simulink model "EV_sim_model"  (R2024a)
settings: Solver=FixedStepAuto  StartTime=0.0  StopTime=time  FixedStep=0.01  RelTol=1e-3
undefined symbols (not defined in the file): Af, Bl, C, Cd, eff_b, eff_g, eff_m, g, GR, Grd, i, Jgb, Jw, L_range, M, pho_air, R_w, U_bat, U_pack
libraries: autolibshared x4
settings Model: Creator=Roshan_PC  LastModifiedBy=Roshan_PC
settings SolverCC: ZeroCrossAlgorithm=Adaptive
settings DebuggingCC: MaskedZcDiagnostic=none  IgnoredZcDiagnostic=none

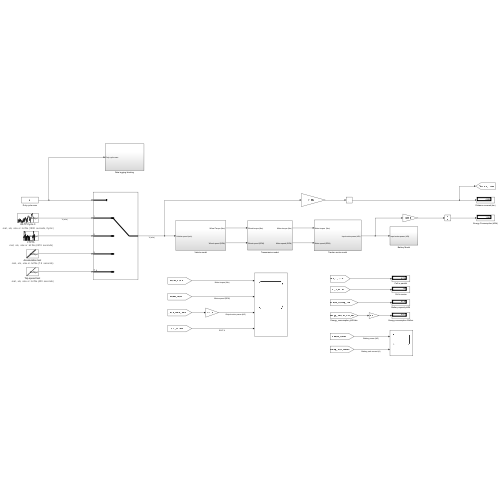
[thumbnail: Simulink's stored preview of the top-level diagram]
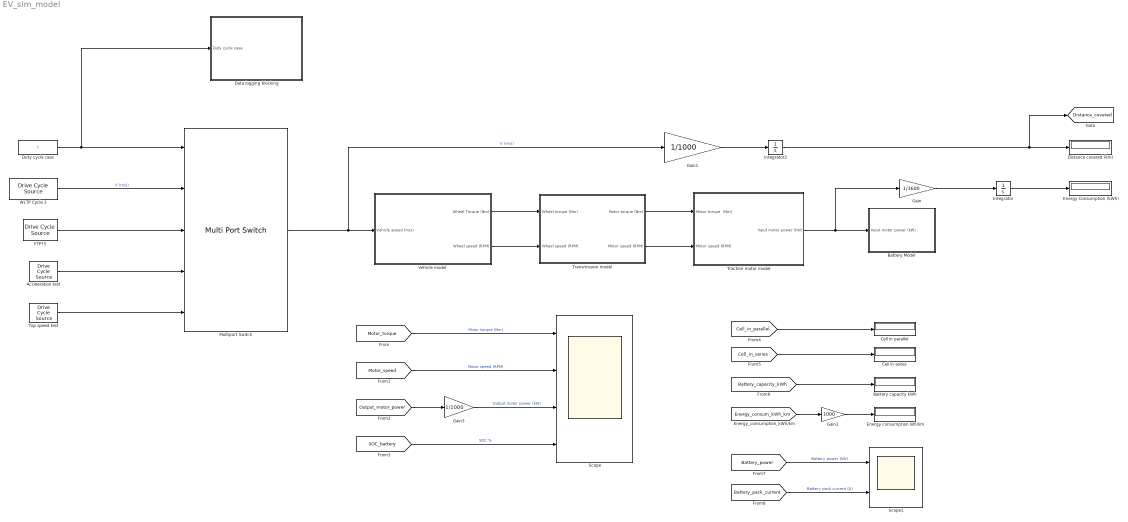
== system EV_sim_model ==
  Acceleration test : autolibshared/Drive Cycle Source  cycleVar=.mat, .xls, .xlsx or .txt file  fileVar=D:\Creation stuff\Academic\MATLAB practice\1_EV_car_system_simulation\Backward_approach\Model-2\Acceleration_Drive_Cycle.xlsx  tfinal="7.9  seconds"  cycleRepeat=off  outAccPort=off  outGearPort=off  gearList=No gear data  t_wot1=5  xdot_woto=0  xdot_wot1=30  t_wot2=20  xdot_wot2=0  t_wotend=30  srcUnit=km/hr  outUnit=m/s  srcAccUnit=m/s/s  outAccUnit=m/s^2  dt=0  aMode=1  faultOption=off  velBnd=2  velBndUnit=mph  inUnit=m/s  timeBnd=1  failOption=off  stopSim=off  maxFaultCnt=10  maxFaultTime=2  maxTotFaultTime=15  traceOption=off  dtTrace=1  traceWindow=10  lastDCname=Custom Data Set  lastOutUnit=mph  lastDT=0  lastTB=1  lastSB=2  forceCalcBound=off
  Battery Model : Subsystem
  Battery capacity kWh : Display
  Cell in parallel : Display
  Cell in series : Display
  Data logging blocking : Subsystem
  Distance covered (km) : Display
  Duty cycle case : Constant  Value=i
  Energy Consumption (kWh) : Display
  Energy consumption Wh/km : Display
  FTP75 : autolibshared/Drive Cycle Source  cycleVar=.mat, .xls, .xlsx or .txt file  fileVar=cycleFTP75.mat  tfinal="2474  seconds"  cycleRepeat=off  outAccPort=off  outGearPort=off  gearList=No gear data  t_wot1=5  xdot_woto=0  xdot_wot1=30  t_wot2=20  xdot_wot2=0  t_wotend=30  srcUnit=m/s  outUnit=m/s  srcAccUnit=m/s/s  outAccUnit=m/s^2  dt=0  aMode=1  faultOption=off  velBnd=2  velBndUnit=mph  inUnit=m/s  timeBnd=1  failOption=off  stopSim=off  maxFaultCnt=10  maxFaultTime=2  maxTotFaultTime=15  traceOption=off  dtTrace=1  traceWindow=10  lastDCname=Custom Data Set 1  lastOutUnit=mph  lastDT=0  lastTB=1  lastSB=2  forceCalcBound=off
  Gain : Gain  Gain=1/3600
  Gain1 : Gain  Gain=1/1000
  Gain2 : Gain  Gain=1000
  Gain3 : Gain  Gain=1/1000
  Integrator : Integrator
  Integrator2 : Integrator
  Multiport Switch : MultiPortSwitch  Inputs=4  RndMeth=Nearest  SaturateOnIntegerOverflow=off  InputSameDT=off
  Scope : Scope  NumInputPorts=4
  Scope1 : Scope  NumInputPorts=2
  Top speed test : autolibshared/Drive Cycle Source  cycleVar=.mat, .xls, .xlsx or .txt file  fileVar=D:\Creation stuff\Academic\MATLAB practice\1_EV_car_system_simulation\Backward_approach\Model-2\Top_speed_drive_cycle.xlsx  tfinal="400  seconds"  cycleRepeat=off  outAccPort=off  outGearPort=off  gearList=No gear data  t_wot1=5  xdot_woto=0  xdot_wot1=30  t_wot2=20  xdot_wot2=0  t_wotend=30  srcUnit=km/hr  outUnit=m/s  srcAccUnit=m/s/s  outAccUnit=m/s^2  dt=0  aMode=1  faultOption=off  velBnd=2  velBndUnit=mph  inUnit=m/s  timeBnd=1  failOption=off  stopSim=off  maxFaultCnt=10  maxFaultTime=2  maxTotFaultTime=15  traceOption=off  dtTrace=1  traceWindow=10  lastDCname=Custom Data Set  lastOutUnit=mph  lastDT=0  lastTB=1  lastSB=2  forceCalcBound=off
  Traction motor model : Subsystem
  Transmission model : Subsystem
  Vehicle model : Subsystem
  WLTP Cycle 3 : autolibshared/Drive Cycle Source  cycleVar=.mat, .xls, .xlsx or .txt file  fileVar=D:\Creation stuff\Academic\MATLAB practice\1_EV_car_system_simulation\Backward_approach\Model-2\WLTC_DRIVE_CYCLE_CLASS_3.xlsx  tfinal="1800  seconds, Cyclic"  cycleRepeat=on  outAccPort=off  outGearPort=off  gearList=No gear data  t_wot1=5  xdot_woto=0  xdot_wot1=30  t_wot2=20  xdot_wot2=0  t_wotend=30  srcUnit=km/hr  outUnit=m/s  srcAccUnit=m/s/s  outAccUnit=m/s^2  dt=0  aMode=1  faultOption=off  velBnd=2  velBndUnit=mph  inUnit=m/s  timeBnd=1  failOption=off  stopSim=off  maxFaultCnt=10  maxFaultTime=2  maxTotFaultTime=15  traceOption=off  dtTrace=1  traceWindow=10  lastDCname=Custom Data Set  lastOutUnit=mph  lastDT=0  lastTB=1  lastSB=2  forceCalcBound=off
  tag scope: Distance_covered=global
  wires:
  Multiport Switch/1 -> Gain1/1, Vehicle model/1(Vehicle speed (m/s))  "V (m/s)"
  Vehicle model/1(Wheel Torque (Nm)) -> Transmission model/1(Wheel torque (Nm))
  Vehicle model/2(Wheel speed (RPM)) -> Transmission model/2(Wheel speed (RPM))
  Transmission model/1(Motor torque (Nm)) -> Traction motor model/1(Motor torque  (Nm))
  Transmission model/2(Motor speed (RPM)) -> Traction motor model/2(Motor speed (RPM))
  Traction motor model/1(Input motor power (kW)) -> Gain/1, Battery Model/1(Input motor power (kW))
  [Battery_pack_current] -> Scope1/2  "Battery pack current (A)"
  [Battery_power] -> Scope1/1  "Battery power (kW)"
  Gain2/1 -> Energy consumption Wh/km/1
  [Cell_in_series] -> Cell in series/1
  [Cell_in_parallel] -> Cell in parallel/1
  [Energy_consum_kWh_km] -> Gain2/1
  [Battery_capacity_kWh] -> Battery capacity kWh/1
  [Motor_torque] -> Scope/1  "Motor torque (Nm)"
  [Motor_speed] -> Scope/2  "Motor speed (RPM)"
  [Output_motor_power] -> Gain3/1
  [SOC_battery] -> Scope/4  "SOC %"
  Integrator/1 -> Energy Consumption (kWh)/1
  Gain/1 -> Integrator/1
  Integrator2/1 -> Distance covered (km)/1, [Distance_covered]
  Gain1/1 -> Integrator2/1
  WLTP Cycle 3/1 -> Multiport Switch/2  "V (m/s)"
  Duty cycle case/1 -> Data logging blocking/1("Duty cycle case "), Multiport Switch/1
  Top speed test/1 -> Multiport Switch/5
  FTP75/1 -> Multiport Switch/3
  Acceleration test/1 -> Multiport Switch/4
  Gain3/1 -> Scope/3  "Output motor power (kW)"

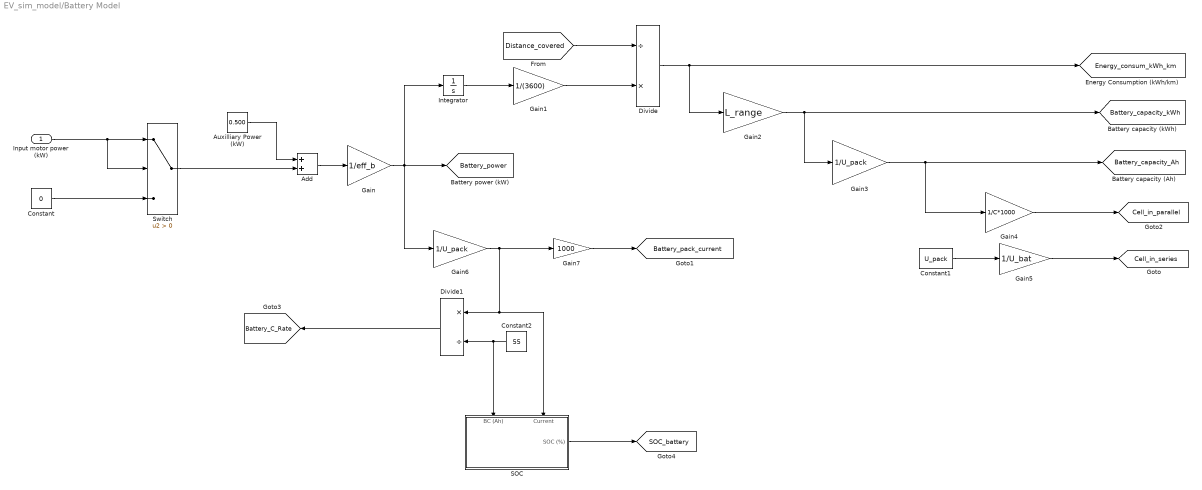
== system EV_sim_model/Battery Model ==
  Input motor power (kW) : Inport
  Add : Sum
  Auxilliary Power (kW) : Constant  Value=0.500
  Constant : Constant  Value=0
  Constant1 : Constant  Value=U_pack
  Constant2 : Constant  Value=55
  Divide : Product  Inputs=/*
  Divide1 : Product  Inputs=*/
  Gain : Gain  Gain=1/eff_b
  Gain1 : Gain  Gain=1/(3600)
  Gain2 : Gain  Gain=L_range
  Gain3 : Gain  Gain=1/U_pack
  Gain4 : Gain  Gain=1/C*1000
  Gain5 : Gain  Gain=1/U_bat
  Gain6 : Gain  Gain=1/U_pack
  Gain7 : Gain  Gain=1000
  Integrator : Integrator
  SOC : Subsystem
      settings: PortSchema="{\"entries\":[{\"content\":{\"sides\":[{\"content\":{},\"type\":\"ConnectorPlacement.EquallySpacedRectSide\",\"uuid\":\"0985c93a-0d74-42c2-8982-61905e894fc7\"},{\"content\":{\"connectorIds\":[\"Out1\"],\"side\":\"RIGHT\"},\"type\":\"ConnectorPlacement.EquallySpacedRectSide\",\"uuid\":\"47ea0ea1-b0a1-43bd-8778-8213b2a428b9\"},{\"content\":{\"connectorIds\":[\"In1\",\"In2\"],\"side\":\"TOP\"},\"type\":\"ConnectorPlacement.EquallySpacedRectSide\",\"uuid\":\"c3724bbf-48db-4247-9168-29f4733f8fd8\"}]},\"type\":\"ConnectorPlacement.EquallySpacedConnector\",\"uuid\":\"539dcac8-68dc-4377-abe5-cb667d6e7e4f\"}],\"packageUris\":[\"http://schema.mathworks.com/mf0/Connector/R2020b\"],\"version\":\"1.0\"}"
  Switch : Switch  Criteria=u2 > Threshold  SaturateOnIntegerOverflow=off  InputSameDT=off
  tag scope: Battery_C_Rate=global, Battery_capacity_Ah=global, Battery_capacity_kWh=global, Battery_pack_current=global, Battery_power=global, Cell_in_parallel=global, Cell_in_series=global, Energy_consum_kWh_km=global, SOC_battery=global
  wires:
  Input motor power (kW)/1 -> Switch/2, Switch/1
  Constant/1 -> Switch/3
  Gain/1 -> [Battery_power], Gain6/1, Integrator/1
  Integrator/1 -> Gain1/1
  Gain1/1 -> Divide/2
  [Distance_covered] -> Divide/1
  Divide/1 -> [Energy_consum_kWh_km], Gain2/1
  Gain2/1 -> Gain3/1, [Battery_capacity_kWh]
  Gain3/1 -> Gain4/1, [Battery_capacity_Ah]
  Gain4/1 -> [Cell_in_parallel]
  Constant1/1 -> Gain5/1
  Gain5/1 -> [Cell_in_series]
  Gain6/1 -> SOC/2(Current), Divide1/1, Gain7/1
  Constant2/1 -> SOC/1(BC (Ah)), Divide1/2
  Divide1/1 -> [Battery_C_Rate]
  SOC/1(SOC (%)) -> [SOC_battery]
  Gain7/1 -> [Battery_pack_current]
  Auxilliary Power (kW)/1 -> Add/1
  Switch/1 -> Add/2
  Add/1 -> Gain/1

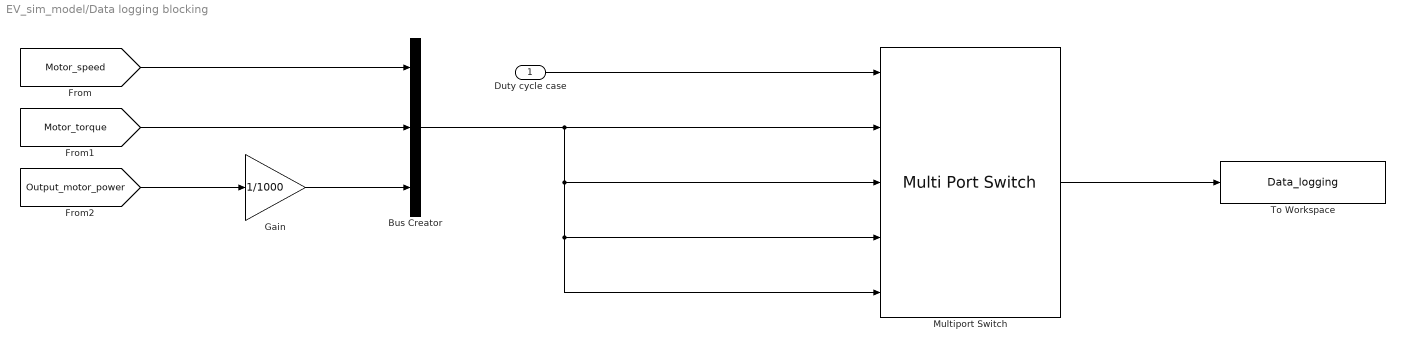
== system EV_sim_model/Data logging blocking ==
  "Duty cycle case " : Inport
  Bus Creator : BusCreator  Inputs=3
  Gain : Gain  Gain=1/1000
  Multiport Switch : MultiPortSwitch  Inputs=4  SaturateOnIntegerOverflow=off  InputSameDT=off
  To Workspace : ToWorkspace  VariableName=Data_logging  SampleTime=-1
      settings: Save2DSignal=2-D array (concatenate along first dimension)
  wires:
  "Duty cycle case "/1 -> Multiport Switch/1
  [Motor_speed] -> Bus Creator/1
  [Motor_torque] -> Bus Creator/2
  [Output_motor_power] -> Gain/1
  Bus Creator/1 -> Multiport Switch/4, Multiport Switch/5, Multiport Switch/3, Multiport Switch/2
  Multiport Switch/1 -> To Workspace/1
  Gain/1 -> Bus Creator/3

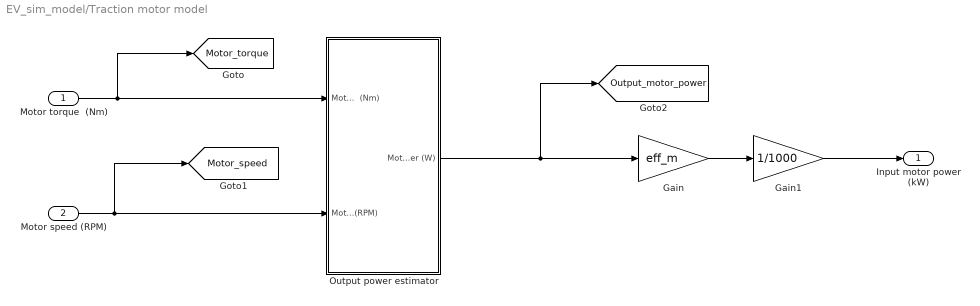
== system EV_sim_model/Traction motor model ==
  Motor torque  (Nm) : Inport
  Motor speed (RPM) : Inport  Port=2
  Gain : Gain  Gain=eff_m
  Gain1 : Gain  Gain=1/1000
  Output power estimator : Subsystem
  Input motor power (kW) : Outport
  tag scope: Motor_speed=global, Motor_torque=global, Output_motor_power=global
  wires:
  Motor torque  (Nm)/1 -> Output power estimator/1(Motor torque  (Nm)), [Motor_torque]
  Motor speed (RPM)/1 -> Output power estimator/2(Motor speed (RPM)), [Motor_speed]
  Output power estimator/1(Motor output power (W)) -> Gain/1, [Output_motor_power]
  Gain/1 -> Gain1/1
  Gain1/1 -> Input motor power (kW)/1

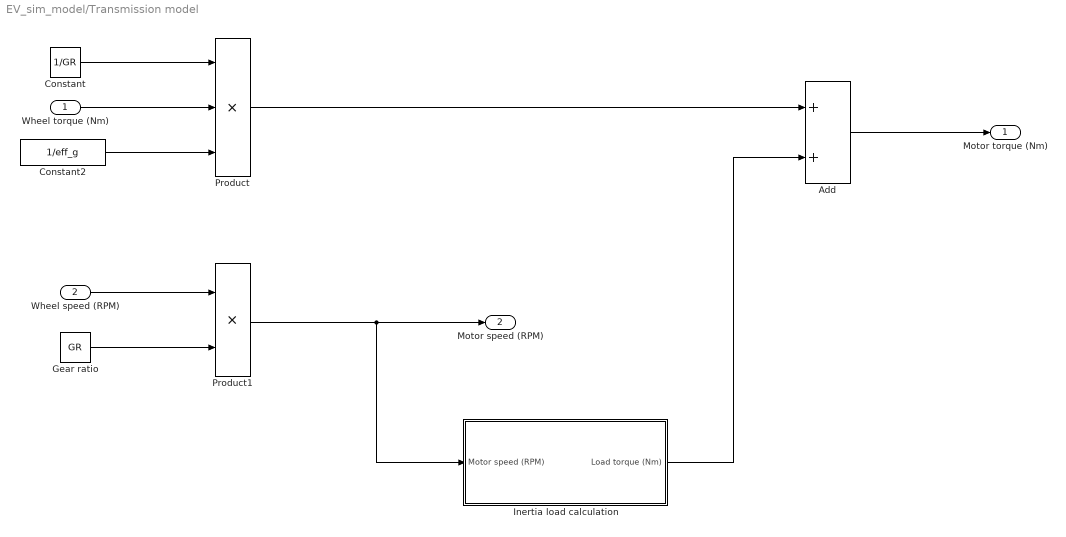
== system EV_sim_model/Transmission model ==
  Wheel torque (Nm) : Inport
  Wheel speed (RPM) : Inport  Port=2
  Add : Sum
  Constant : Constant  Value=1/GR
  Constant2 : Constant  Value=1/eff_g
  Gear ratio : Constant  Value=GR
  Inertia load calculation : Subsystem
  Product : Product  Inputs=3
  Product1 : Product
  Motor torque (Nm) : Outport
  Motor speed (RPM) : Outport  Port=2
  wires:
  Constant/1 -> Product/1
  Wheel torque (Nm)/1 -> Product/2
  Wheel speed (RPM)/1 -> Product1/1
  Gear ratio/1 -> Product1/2
  Product1/1 -> Inertia load calculation/1(Motor speed (RPM)), Motor speed (RPM)/1
  Constant2/1 -> Product/3
  Product/1 -> Add/1
  Add/1 -> Motor torque (Nm)/1
  Inertia load calculation/1(Load torque (Nm)) -> Add/2

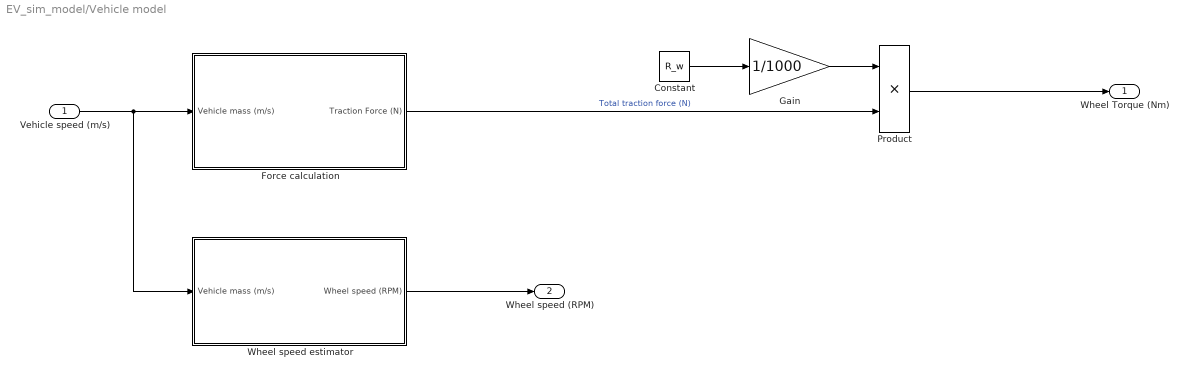
== system EV_sim_model/Vehicle model ==
  Vehicle speed (m/s) : Inport
  Constant : Constant  Value=R_w
  Force calculation : Subsystem
  Gain : Gain  Gain=1/1000
  Product : Product
  Wheel speed estimator : Subsystem
  Wheel Torque (Nm) : Outport
  Wheel speed (RPM) : Outport  Port=2
  wires:
  Vehicle speed (m/s)/1 -> Wheel speed estimator/1(Vehicle mass (m/s)), Force calculation/1(Vehicle mass (m/s))
  Wheel speed estimator/1(Wheel speed (RPM)) -> Wheel speed (RPM)/1
  Gain/1 -> Product/1
  Product/1 -> Wheel Torque (Nm)/1
  Constant/1 -> Gain/1
  Force calculation/1(Traction Force (N)) -> Product/2  "Total traction force (N)"

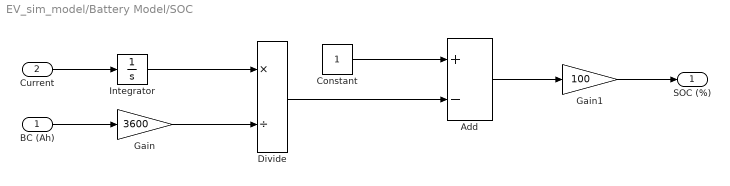
== system EV_sim_model/Battery Model/SOC ==
  BC (Ah) : Inport
  Current : Inport  Port=2
  Add : Sum  Inputs=+-
  Constant : Constant
  Divide : Product  Inputs=*/
  Gain : Gain  Gain=3600
  Gain1 : Gain  Gain=100
  Integrator : Integrator
  SOC (%) : Outport
  wires:
  Current/1 -> Integrator/1
  Integrator/1 -> Divide/1
  BC (Ah)/1 -> Gain/1
  Gain/1 -> Divide/2
  Constant/1 -> Add/1
  Divide/1 -> Add/2
  Add/1 -> Gain1/1
  Gain1/1 -> SOC (%)/1

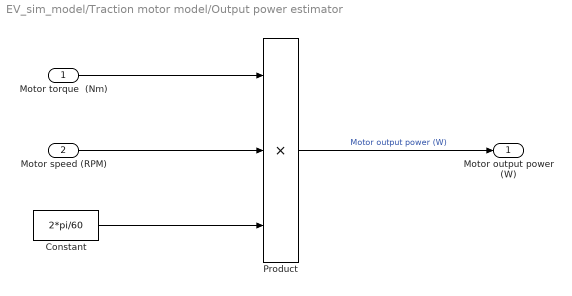
== system EV_sim_model/Traction motor model/Output power estimator ==
  Motor torque  (Nm) : Inport
  Motor speed (RPM) : Inport  Port=2
  Constant : Constant  Value=2*pi/60
  Product : Product  Inputs=3
  Motor output power (W) : Outport
  wires:
  Constant/1 -> Product/3
  Motor speed (RPM)/1 -> Product/2
  Motor torque  (Nm)/1 -> Product/1
  Product/1 -> Motor output power (W)/1  "Motor output power (W)"

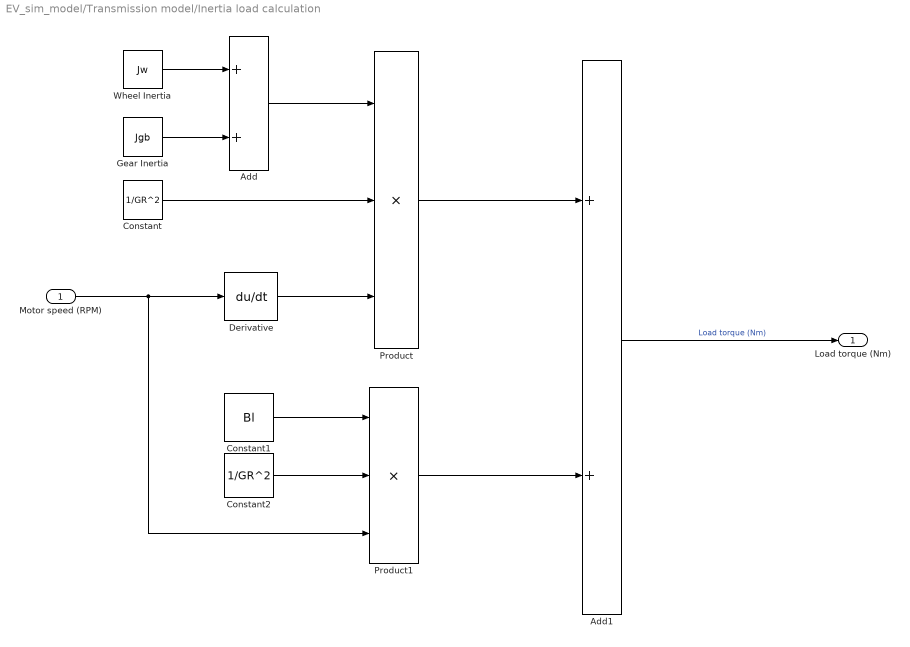
== system EV_sim_model/Transmission model/Inertia load calculation ==
  Motor speed (RPM) : Inport
  Add : Sum
  Add1 : Sum
  Constant : Constant  Value=1/GR^2
  Constant1 : Constant  Value=Bl
  Constant2 : Constant  Value=1/GR^2
  Derivative : Derivative
  Gear Inertia : Constant  Value=Jgb
  Product : Product  Inputs=3
  Product1 : Product  Inputs=3
  Wheel Inertia : Constant  Value=Jw
  Load torque (Nm) : Outport
  wires:
  Wheel Inertia/1 -> Add/1
  Gear Inertia/1 -> Add/2
  Add/1 -> Product/1
  Constant/1 -> Product/2
  Motor speed (RPM)/1 -> Product1/3, Derivative/1
  Derivative/1 -> Product/3
  Constant1/1 -> Product1/1
  Constant2/1 -> Product1/2
  Product1/1 -> Add1/2
  Product/1 -> Add1/1
  Add1/1 -> Load torque (Nm)/1  "Load torque (Nm)"

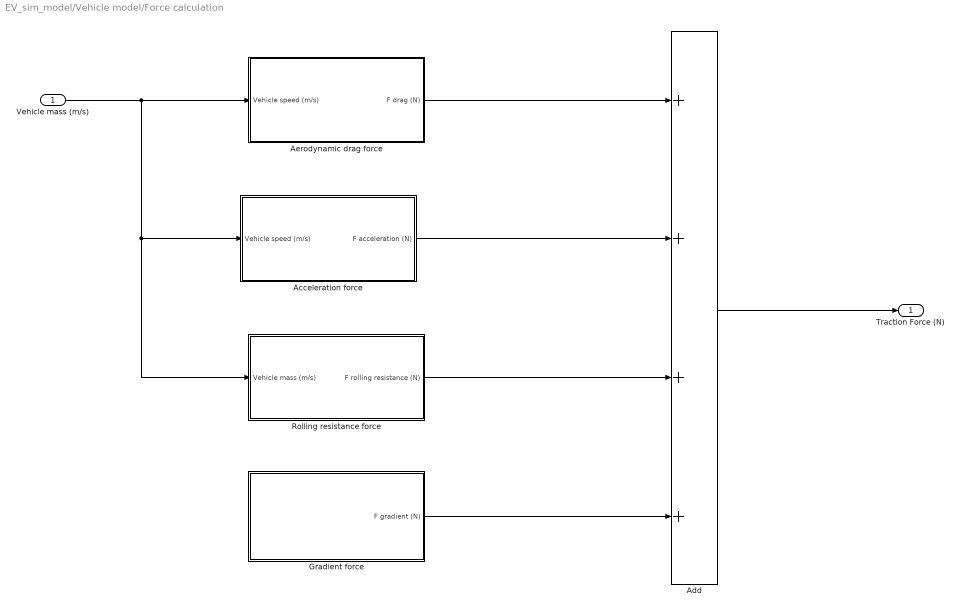
== system EV_sim_model/Vehicle model/Force calculation ==
  Vehicle mass (m/s) : Inport
  Acceleration force : Subsystem
  Add : Sum  Inputs=++++
  Aerodynamic drag force : Subsystem
  Gradient force : Subsystem
  Rolling resistance force : Subsystem
  Traction Force (N) : Outport
  wires:
  Acceleration force/1(F acceleration (N)) -> Add/2
  Vehicle mass (m/s)/1 -> Rolling resistance force/1(Vehicle mass (m/s)), Acceleration force/1(Vehicle speed (m/s)), Aerodynamic drag force/1(Vehicle speed (m/s))
  Aerodynamic drag force/1(F drag (N)) -> Add/1
  Gradient force/1(F gradient (N)) -> Add/4
  Rolling resistance force/1(F rolling resistance (N)) -> Add/3
  Add/1 -> Traction Force (N)/1

== system EV_sim_model/Vehicle model/Wheel speed estimator ==
  Vehicle mass (m/s) : Inport
  Gain : Gain  Gain=60/(R_w/1000*2*pi)
  Wheel speed (RPM) : Outport
  wires:
  Vehicle mass (m/s)/1 -> Gain/1
  Gain/1 -> Wheel speed (RPM)/1

== system EV_sim_model/Vehicle model/Force calculation/Acceleration force ==
  Vehicle speed (m/s) : Inport
  Derivative : Derivative
  Product : Product
  Vehicle mass : Constant  Value=M
  F acceleration (N) : Outport
  wires:
  Vehicle speed (m/s)/1 -> Derivative/1
  Derivative/1 -> Product/1
  Product/1 -> F acceleration (N)/1
  Vehicle mass/1 -> Product/2

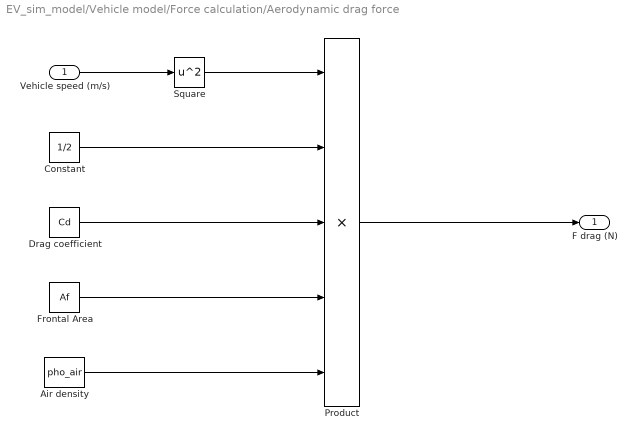
== system EV_sim_model/Vehicle model/Force calculation/Aerodynamic drag force ==
  Vehicle speed (m/s) : Inport
  Air density : Constant  Value=pho_air
  Constant : Constant  Value=1/2
  Drag coefficient : Constant  Value=Cd
  Frontal Area : Constant  Value=Af
  Product : Product  Inputs=5
  Square : Math  Operator=square
  F drag (N) : Outport
  wires:
  Vehicle speed (m/s)/1 -> Square/1
  Square/1 -> Product/1
  Constant/1 -> Product/2
  Drag coefficient/1 -> Product/3
  Frontal Area/1 -> Product/4
  Air density/1 -> Product/5
  Product/1 -> F drag (N)/1

== system EV_sim_model/Vehicle model/Force calculation/Gradient force ==
  Constant : Constant  Value=sin(Grd)
  Product : Product
  Vehicle mass (kg) : Constant  Value=M
  g : Gain  Gain=g
  F gradient (N) : Outport
  wires:
  Vehicle mass (kg)/1 -> g/1
  g/1 -> Product/1
  Constant/1 -> Product/2
  Product/1 -> F gradient (N)/1

== system EV_sim_model/Vehicle model/Force calculation/Rolling resistance force ==
  Vehicle mass (m/s) : Inport
  Product : Product
  Rolling resistance coefficient estimator : Subsystem
  Vehicle mass : Constant  Value=M
  F rolling resistance (N) : Outport
  wires:
  Vehicle mass/1 -> Product/2
  Product/1 -> F rolling resistance (N)/1
  Rolling resistance coefficient estimator/1(Cr) -> Product/1
  Vehicle mass (m/s)/1 -> Rolling resistance coefficient estimator/1(V (m/s))

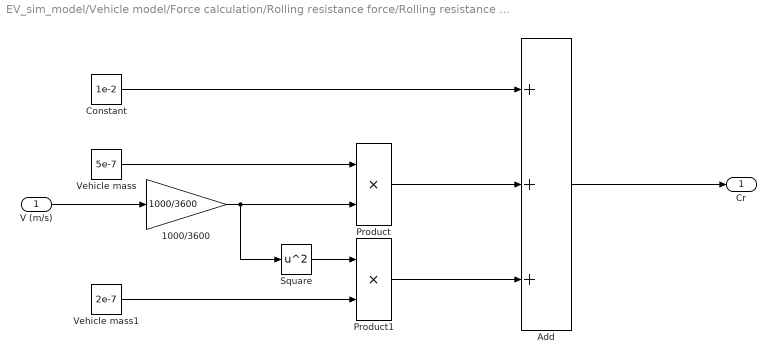
== system EV_sim_model/Vehicle model/Force calculation/Rolling resistance force/Rolling resistance coefficient estimator ==
  V (m/s) : Inport
  1000/3600 : Gain  Gain=1000/3600
  Add : Sum  Inputs=+++
  Constant : Constant  Value=1e-2
  Product : Product
  Product1 : Product
  Square : Math  Operator=square
  Vehicle mass : Constant  Value=5e-7
  Vehicle mass1 : Constant  Value=2e-7
  Cr : Outport
  wires:
  V (m/s)/1 -> 1000/3600/1
  Constant/1 -> Add/1
  Vehicle mass/1 -> Product/1
  1000/3600/1 -> Product/2, Square/1
  Product/1 -> Add/2
  Vehicle mass1/1 -> Product1/2
  Square/1 -> Product1/1
  Product1/1 -> Add/3
  Add/1 -> Cr/1
